simulink model "double_integrator_Constraint_Lifting"  (R2024a)
settings: Solver=ode4  StartTime=0.0  StopTime=20  FixedStep=0.1  RelTol=1e-3
settings Model: Creator=PhDstudent1  LastModifiedBy=NITRO5
settings DebuggingCC: UnderSpecifiedDimensionMsg=warning

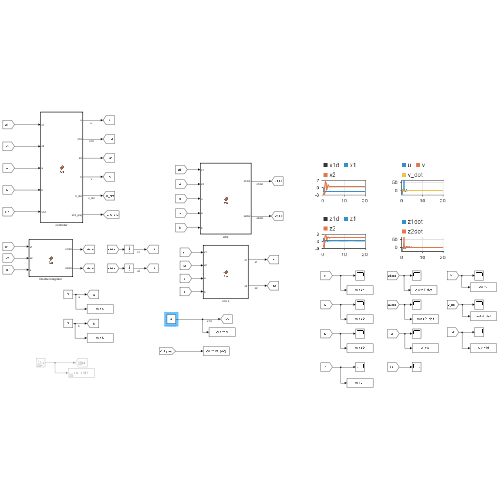
[thumbnail: Simulink's stored preview of the top-level diagram]
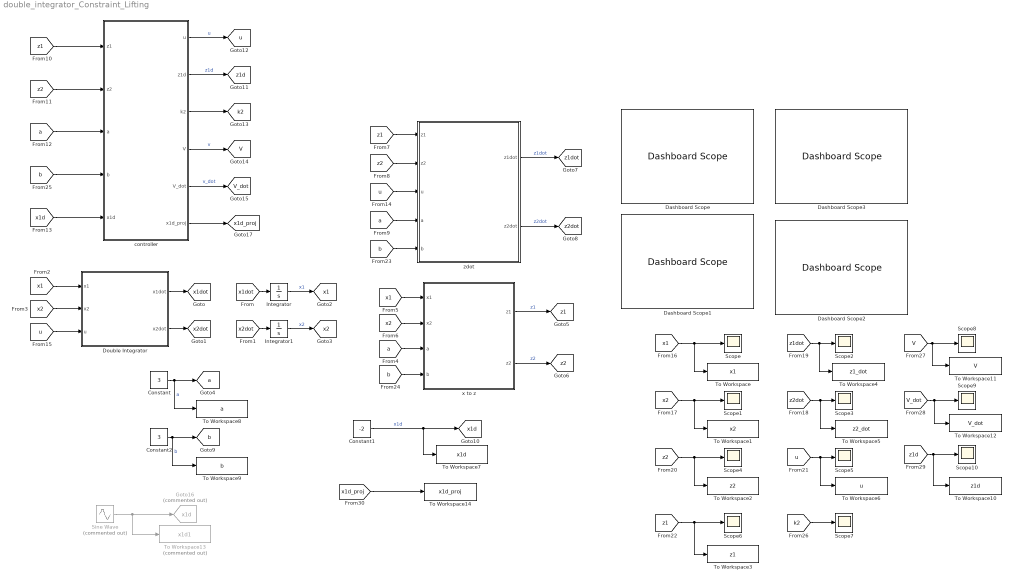
== system double_integrator_Constraint_Lifting ==
  Constant : Constant  Value=3
  Constant1 : Constant  Value=-2
  Constant2 : Constant  Value=3
  Dashboard Scope{,1..3} (4 alike) : DashboardScope
  Double Integrator : MATLAB Function  TreatAsAtomicUnit=on
  Goto16 : Goto  Commented=on  GotoTag=x1d  TagVisibility=global
  Integrator : Integrator
  Integrator1 : Integrator
  Scope{,1..10} (11 alike) : Scope
  Sine Wave : Sin  Commented=on  SampleTime=0
  To Workspace : ToWorkspace  VariableName=x1  SaveFormat=Timeseries  SampleTime=-1
  To Workspace1 : ToWorkspace  VariableName=x2  SaveFormat=Timeseries  SampleTime=-1
  To Workspace10 : ToWorkspace  VariableName=z1d  SaveFormat=Timeseries  SampleTime=-1
  To Workspace11 : ToWorkspace  VariableName=V  SaveFormat=Timeseries  SampleTime=-1
  To Workspace12 : ToWorkspace  VariableName=V_dot  SaveFormat=Timeseries  SampleTime=-1
  To Workspace13 : ToWorkspace  Commented=on  VariableName=x1d1  SaveFormat=Timeseries  SampleTime=-1
  To Workspace14 : ToWorkspace  VariableName=x1d_proj  SaveFormat=Timeseries  SampleTime=-1
  To Workspace2 : ToWorkspace  VariableName=z2  SaveFormat=Timeseries  SampleTime=-1
  To Workspace3 : ToWorkspace  VariableName=z1  SaveFormat=Timeseries  SampleTime=-1
  To Workspace4 : ToWorkspace  VariableName=z1_dot  SaveFormat=Timeseries  SampleTime=-1
  To Workspace5 : ToWorkspace  VariableName=z2_dot  SaveFormat=Timeseries  SampleTime=-1
  To Workspace6 : ToWorkspace  VariableName=u  SaveFormat=Timeseries  SampleTime=-1
  To Workspace7 : ToWorkspace  VariableName=x1d  SaveFormat=Timeseries  SampleTime=-1
  To Workspace8 : ToWorkspace  VariableName=a  SaveFormat=Timeseries  SampleTime=-1
  To Workspace9 : ToWorkspace  VariableName=b  SaveFormat=Timeseries  SampleTime=-1
  controller : MATLAB Function  TreatAsAtomicUnit=on
  x to z : MATLAB Function  TreatAsAtomicUnit=on
  zdot : MATLAB Function  TreatAsAtomicUnit=on
  tag scope: V=global, V_dot=global, a=global, b=global, k2=global, u=global, x1=global, x1d=global, x1d_proj=global, x1dot=global, x2=global, x2dot=global, z1=global, z1d=global, z1dot=global, z2=global, z2dot=global
  wires:
  Double Integrator/1(x1dot) -> [x1dot]
  Double Integrator/2(x2dot) -> [x2dot]
  [x1dot] -> Integrator/1
  [x2dot] -> Integrator1/1
  Integrator/1 -> [x1]  "x1"
  Integrator1/1 -> [x2]  "x2"
  [x1] -> Double Integrator/1(x1)
  [x2] -> Double Integrator/2(x2)
  Constant/1 -> To Workspace8/1, [a]  "a"
  [a] -> x to z/3(a)
  [x1] -> x to z/1(x1)
  [x2] -> x to z/2(x2)
  x to z/1(z1) -> [z1]  "z1"
  x to z/2(z2) -> [z2]  "z2"
  [z1] -> zdot/1(z1)
  [z2] -> zdot/2(z2)
  [a] -> zdot/4(a)
  zdot/2(z2dot) -> [z2dot]  "z2dot"
  zdot/1(z1dot) -> [z1dot]  "z1dot"
  [z1] -> controller/1(z1)
  [a] -> controller/3(a)
  Constant1/1 -> [x1d], To Workspace7/1  "x1d"
  [x1d] -> controller/5(x1d)
  controller/2(z1d) -> [z1d]  "z1d"
  [u] -> zdot/3(u)
  [u] -> Double Integrator/3(u)
  [x1] -> To Workspace/1, Scope/1
  [x2] -> To Workspace1/1, Scope1/1
  [z2dot] -> To Workspace5/1, Scope3/1
  [z1dot] -> To Workspace4/1, Scope2/1
  [z2] -> To Workspace2/1, Scope4/1
  [u] -> To Workspace6/1, Scope5/1
  controller/1(u) -> [u]  "u"
  [z1] -> To Workspace3/1, Scope6/1
  [z2] -> controller/2(z2)
  Constant2/1 -> To Workspace9/1, [b]  "b"
  [b] -> zdot/5(b)
  [b] -> x to z/4(b)
  [b] -> controller/4(b)
  controller/3(k2) -> [k2]
  [k2] -> Scope7/1
  controller/4(V) -> [V]  "v"
  [V] -> To Workspace11/1, Scope8/1
  controller/5(V_dot) -> [V_dot]  "v_dot"
  [V_dot] -> To Workspace12/1, Scope9/1
  [z1d] -> To Workspace10/1, Scope10/1
  Sine Wave/1 -> To Workspace13/1, Goto16/1
  controller/6(x1d_proj) -> [x1d_proj]
  [x1d_proj] -> To Workspace14/1

== matlab function double_integrator_Constraint_Lifting/x to z ==
  data: x1 input; z1 output; x2 input; a input; z2 output; b input
function [z1,z2] = fcn(x1,x2,a,b)
z1 = a*atanh(x1/a);
z2 = b*atanh(x2/b);
end

== matlab function double_integrator_Constraint_Lifting/Double Integrator ==
  data: x1 input; x2 input; u input; x1dot output; x2dot output
function [x1dot,x2dot] = fcn(x1,x2,u)
x1dot = x2;
x2dot = u;
end

== matlab function double_integrator_Constraint_Lifting/zdot ==
  data: z1 input; z2 input; u input; z1dot output; a input; z2dot output; b input
function [z1dot,z2dot] = fcn(z1,z2,u,a,b)
z1dot = (cosh(z1/a)^2)*(b*tanh(z2/b));
z2dot = (cosh(z2/b)^2)*u;
end

== matlab function double_integrator_Constraint_Lifting/controller ==
  data: u output; z1 input; z2 input; a input; b input; x1d input; z1d output; k2 output; V output; V_dot output; x1d_proj output

function [u,z1d,k2,V,V_dot,x1d_proj] = fcn(z1,z2,a,b,x1d)
k1 = 10;
k2 = 1/k1;

epsilon = 1e-2;
if (abs(x1d) >= abs(a))
    x1d_proj = min(max(x1d,-a + epsilon),a - epsilon);
else
    x1d_proj = x1d;
end
z1d = a*atanh(x1d_proj/a);

e1 = z1 - z1d;
z2d = -k1*e1;

e2 = (cosh(z1/a)^2)*(b*tanh(z2/b)) - z2d;
% inv_term = (sech(z1/a)^2)*(b^2*cosh(z1/a)^4 - (e2 - k1*e1)^2);
inv_term = sech(z2/b)^2*b^2*cosh(z1/a)^2;

% u = -inv_term*((2/a)*(e2 - k1*e1)^2*tanh(z1/a)*cosh(z2/b)^2 - (2/a)*b^2*cosh(z1/a)^4*tanh(z1/a)*tanh(z2/b)^2*cosh(z2/b)^2 - ((e2 - k1*e1)^2 - b^2*cosh(z1/a)^4)*cosh(z2/b)^2*k2*e2);
u = -inv_term*(k2*e2);
V = 0.5*e1^2 + 0.5*log(cosh(z2/b)^2);
V_dot = -(sqrt(k1)*e1 - sqrt(k2)*e2)^2;
end
